simulink model "vehicle_model"  (R2026a)
settings: Solver=VariableStepAuto  StopTime=30
settings Model: Creator=HP  LastModifiedBy=HP

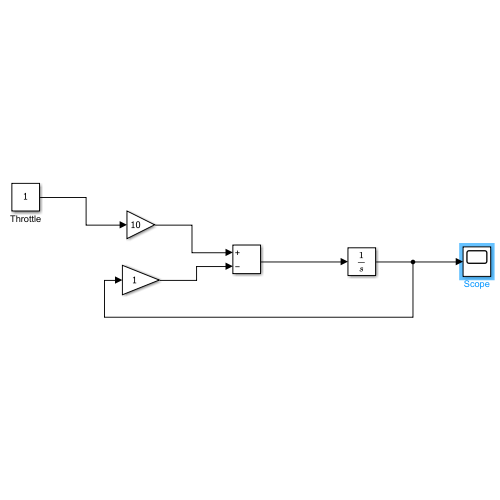
[thumbnail: Simulink's stored preview of the top-level diagram]
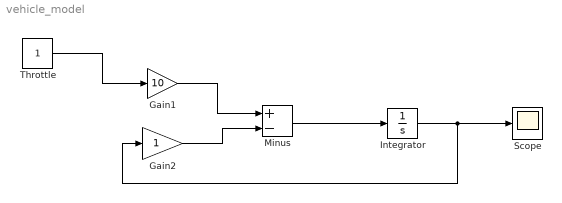
== system vehicle_model ==
  Gain1 : Gain  Gain=10
  Gain2 : Gain
  Integrator : Integrator
  Minus : Sum  Inputs=+-
  Scope : Scope
      settings: ActiveDisplayYMinimum=-202.82132594960632  ActiveDisplayYMaximum=1392.5306271753932
  Throttle : Constant
  wires:
  Minus/1 -> Integrator/1
  Throttle/1 -> Gain1/1
  Gain1/1 -> Minus/1
  Integrator/1 -> Gain2/1, Scope/1
  Gain2/1 -> Minus/2
